simulink model "spmet_realtime"  (R2020a)
settings: Solver=FixedStepDiscrete  StartTime=0.0  StopTime=500  FixedStep=0.01  RelTol=1e-3  EnableMultiTasking=on
undefined symbols (not defined in the file or in its folder): Green, led0
libraries: simulink x1, embdlinuxlib x1
settings Model: Creator=Andreas  LastModifiedBy=Andreas
settings SolverCC: PositivePriorityOrder=on
settings OptimizationCC: EnhancedBackFolding=on  PassReuseOutputArgsAs=Individual arguments  ZeroExternalMemoryAtStartup=off  ZeroInternalMemoryAtStartup=off  MaxStackSize=64  OptimizeBlockOrder=speed  DifferentSizesBufferReuse=on  OptimizationCustomize=off  EfficientTunableParamExpr=on
settings DebuggingCC: ParameterTunabilityLossMsg=error  UnderSpecifiedDimensionMsg=warning
settings HardwareCC: ProdBitPerPointer=32  ProdBitPerSizeT=32  ProdBitPerPtrDiffT=32  ProdLargestAtomicInteger=Long  ProdLargestAtomicFloat=Double  ProdWordSize=32  ProdLongLongMode=on  ProdHWDeviceType=ARM Compatible->ARM Cortex
settings RTWCC: SystemTargetFile=ert.tlc  HardwareBoard=Raspberry Pi  TemplateMakefile=ert_default_tmf  GenerateReport=on  Toolchain=GNU GCC Raspberry Pi  BuildConfiguration=Faster Runs  IncludeHyperlinkInReport=on  LaunchReport=on  GenerateTraceInfo=on  GenerateTraceReport=on  GenerateTraceReportSl=on  GenerateTraceReportSf=on  GenerateTraceReportEml=on
settings CodeAppCC: ForceParamTrailComments=on  IgnoreCustomStorageClasses=off  OperatorAnnotations=on  SimulinkDataObjDesc=on  SFDataObjDesc=on  InsertBlockDesc=on
settings ERTTargetCC: SupportContinuousTime=on  SupportVariableSizeSignals=on

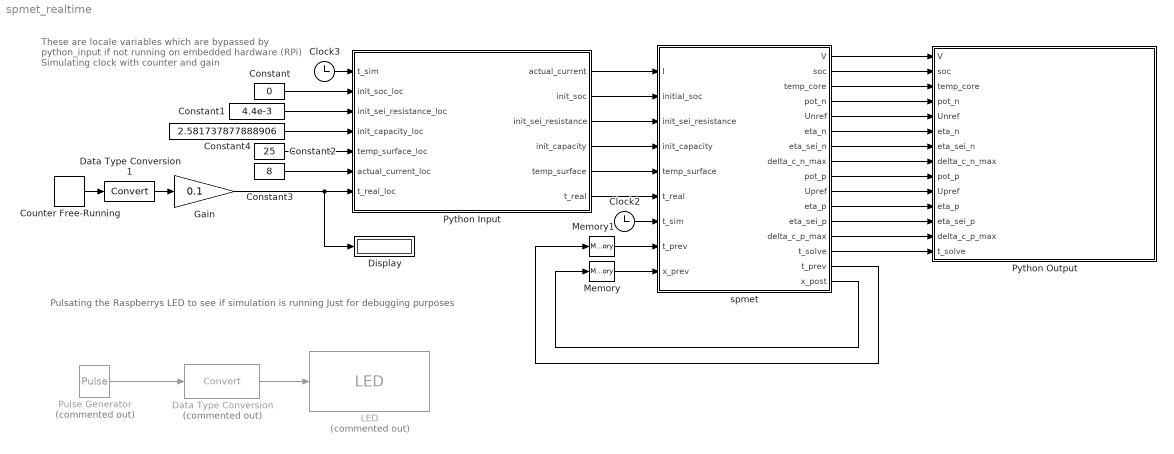
== system spmet_realtime ==
  note: Pulsating the Raspberrys LED to see if simulation is running
      | Just for debugging purposes
  note: These are locale variables
      | which are bypassed by
      | python_input if not running
      | on embedded hardware (RPi)
      |
      |
      |
      |
      |
      |
      |
      |
      | Simulating clock with counter and gain
  Clock2 : Clock
  Clock3 : Clock
  Constant : Constant  Value=0
  Constant1 : Constant  Value=4.4e-3
  Constant2 : Constant  Value=25
  Constant3 : Constant  Value=8
  Constant4 : Constant  Value=2.581737877888906
  Counter Free-Running : simulink/Sources/Counter Free-Running  NumBits=64  tsamp=-1
  Data Type Conversion : DataTypeConversion  Commented=on
  Data Type Conversion1 : DataTypeConversion
  Display : Display
  Gain : Gain  Gain=0.1
  LED : embdlinuxlib/LED  Commented=on  board=Pi 3 Model B+  led=led0 (Green)  blockPlatform=Raspberry Pi
      settings: SourceProductBaseCode=SC_BEAGLEBONE_BLUE,RASPPI
  Memory : Memory
  Memory1 : Memory
  Pulse Generator : DiscretePulseGenerator  Commented=on  PulseType=Time based  Period=4  PulseWidth=50
  Python Input : MATLAB Function  TreatAsAtomicUnit=on
  Python Output : MATLAB Function  TreatAsAtomicUnit=on
  spmet : MATLAB Function  TreatAsAtomicUnit=on
  wires:
  Data Type Conversion/1 -> LED/1
  Pulse Generator/1 -> Data Type Conversion/1
  Clock2/1 -> spmet/7(t_sim)
  Memory/1 -> spmet/9(x_prev)
  Memory1/1 -> spmet/8("t_prev ")
  Clock3/1 -> Python Input/1(t_sim)
  Python Input/2(init_soc) -> spmet/2(initial_soc)
  Python Input/1(actual_current) -> spmet/1(I)
  Constant/1 -> Python Input/2(init_soc_loc)
  Constant3/1 -> Python Input/6(actual_current_loc)
  Data Type Conversion1/1 -> Gain/1
  Counter Free-Running/1 -> Data Type Conversion1/1
  Gain/1 -> Display/1, Python Input/7(t_real_loc)
  spmet/16(x_post) -> Memory/1
  spmet/15(t_prev) -> Memory1/1
  Python Input/5(temp_surface) -> spmet/5(temp_surface)
  Python Input/6(t_real) -> spmet/6(t_real)
  Constant2/1 -> Python Input/5(temp_surface_loc)
  spmet/2(soc) -> Python Output/2(soc)
  spmet/3(temp_core) -> Python Output/3(temp_core)
  spmet/4(pot_n) -> Python Output/4(pot_n)
  spmet/5(Unref) -> Python Output/5(Unref)
  spmet/6(eta_n) -> Python Output/6(eta_n)
  spmet/7(eta_sei_n) -> Python Output/7(eta_sei_n)
  spmet/8(delta_c_n_max) -> Python Output/8(delta_c_n_max)
  spmet/9(pot_p) -> Python Output/9(pot_p)
  spmet/10(Upref) -> Python Output/10(Upref)
  spmet/11(eta_p) -> Python Output/11(eta_p)
  spmet/12(eta_sei_p) -> Python Output/12(eta_sei_p)
  spmet/13(delta_c_p_max) -> Python Output/13(delta_c_p_max)
  spmet/14(t_solve) -> Python Output/14(t_solve)
  spmet/1(V) -> Python Output/1(V)
  Python Input/4(init_capacity) -> spmet/4(init_capacity)
  Python Input/3(init_sei_resistance) -> spmet/3(init_sei_resistance)
  Constant1/1 -> Python Input/3(init_sei_resistance_loc)
  Constant4/1 -> Python Input/4(init_capacity_loc)

== matlab function spmet_realtime/Python Output ==
  data: V input; soc input; temp_core input; pot_n input; Unref input; eta_n input; eta_sei_n input; delta_c_n_max input; pot_p input; Upref input; eta_p input; eta_sei_p input; delta_c_p_max input; t_solve input
function python_output(V, soc, temp_core ,pot_n, Unref, eta_n, eta_sei_n, delta_c_n_max, pot_p, Upref, eta_p, eta_sei_p, delta_c_p_max, t_solve)
 
fprintf(1,"OUT_STRING: V=%f, soc=%f, temp_core=%f, pot_n=%f, Unref=%f, eta_n=%f, eta_sei_n=%f, delta_c_n_max=%f, pot_p=%f, Upref=%f, eta_p=%f, eta_sei_p=%f, delta_c_p_max=%f, t_solve=%f\n"...
            ,V,soc, temp_core, pot_n, Unref, eta_n, eta_sei_n, delta_c_n_max, pot_p, Upref, eta_p, eta_sei_p, delta_c_p_max, t_solve);

end

== matlab function spmet_realtime/Python Input ==
  data: actual_current output; init_soc output; init_sei_resistance output; init_capacity output; temp_surface output; t_sim input; t_real output; init_soc_loc input; init_sei_resistance_loc input; init_capacity_loc input; temp_surface_loc input; actual_current_loc input; t_real_loc input
function [actual_current, init_soc, init_sei_resistance, init_capacity, temp_surface, t_real]...
    =python_input(t_sim, init_soc_loc, init_sei_resistance_loc, init_capacity_loc, temp_surface_loc, actual_current_loc, t_real_loc)

if t_sim==0
    % at start of the Simulation
    
    fprintf(1,"init_soc\n");
    init_soc=0.0; %init
    init_soc=init_soc_loc; %setting to locale value
    coder.ceval('scanf','%lf',coder.ref(init_soc)); % read from stdin
    
    fprintf(1,"init_sei_resistance\n");
    init_sei_resistance=0.0; %init
    init_sei_resistance=init_sei_resistance_loc; %setting to locale value
    coder.ceval('scanf','%lf',coder.ref(init_sei_resistance)); % read from stdin
    
    fprintf(1,"init_capacity\n");
    init_capacity=0.0; %init
    init_capacity=init_capacity_loc; %setting to locale value
    coder.ceval('scanf','%lf',coder.ref(init_capacity)); % read from stdin

    
    % value is not used in first time step but the coder needs it defined
    actual_current=0;
    
else
    % during simulation
    fprintf(1,"actual_current\n");
    actual_current=0.0; %init
    actual_current=actual_current_loc; %setting to locale value
    coder.ceval('scanf','%lf',coder.ref(actual_current)); % read from stdin
    
    % value is not used in during simulation but the coder needs it defined
    init_soc=0;
    init_sei_resistance=0;
    init_capacity=0;

end

% needed in every time step

fprintf(1,"temp_surface\n");
temp_surface=0.0; %init
temp_surface=temp_surface_loc; %setting to locale value
coder.ceval('scanf','%lf',coder.ref(temp_surface)); % read from stdin

fprintf(1,"t_real\n");
t_real=0.0; %init
t_real=t_real_loc; %setting to locale value
coder.ceval('scanf','%lf',coder.ref(t_real)); % read from stdin
end

== matlab function spmet_realtime/spmet ==
  data: V output; soc output; temp_core output; pot_n output; Unref output; eta_n output; eta_sei_n output; delta_c_n_max output; pot_p output; Upref output; eta_p output; eta_sei_p output; delta_c_p_max output; t_solve output; I input; initial_soc input; init_sei_resistance input; init_capacity input; temp_surface input; t_real input; t_sim input; t_prev input; x_prev input; t_prev output; x_post output
function [V, soc, temp_core ,pot_n, Unref, eta_n, eta_sei_n, delta_c_n_max, pot_p, Upref, eta_p, eta_sei_p, delta_c_p_max, t_solve, t_prev, x_post]...
    = spmet(I, initial_soc, init_sei_resistance, init_capacity, temp_surface, t_real, t_sim, t_prev, x_prev)


%% Single Particle Model w/ Electrolyte & Temperature
% Published December 18, 2016 by Professor Scott Moura
% Adapted July 16, 2020 by Matthias Wanzel and Nikolaos Wassiliadis

% addpath(genpath(pwd));

%% Electrochemical model parameter
% Load US18650VTC5A NCA cell parameter
p = params_fn(init_capacity, init_sei_resistance);

%% Initial values for coder
% As the coder (for Simulink) needs to know the dimensions before
% assignment, the constant system matrices have to be defined here

p.ce.M1n = sparse(9,9);
p.ce.M2n = sparse(9,2);
p.ce.M3n = sparse(9,9);
p.ce.M4n = sparse(9,2);
p.ce.M5n = sparse(9,9);

p.ce.M1s = sparse(4,4);
p.ce.M2s = sparse(4,2);
p.ce.M3s = sparse(4,4);
p.ce.M4s = sparse(4,2);
p.ce.M1p = sparse(9,9);
p.ce.M2p = sparse(9,2);
p.ce.M3p = sparse(9,9);
p.ce.M4p = sparse(9,2);
p.ce.M5p = sparse(9,9);

p.ce.C = sparse(4,22);

% Calculate C-Rate
[cn_low,cp_low] = init_SOC(p,0);
[cn_high,cp_high] = init_SOC(p,100); 
Delta_cn = cn_high-cn_low;
Delta_cp = cp_low-cp_high;
qn = p.epsilon_s_n*p.Area*p.L_n*Delta_cn*p.Faraday/3600; 
qp = p.epsilon_s_p*p.Area*p.L_p*Delta_cp*p.Faraday/3600;
p.OneC = min(p.epsilon_s_n*p.L_n*Delta_cn*p.Area*p.Faraday/3600, p.epsilon_s_p*p.L_p*p.Area*Delta_cp*p.Faraday/3600);

%% Use one Input Value
% Live calculation based on Simulink input

if t_sim==0
    t_prev=t_real;
end

t_intermediate = (t_prev+t_real)/2;

t = [t_prev, t_intermediate, t_real];
I = I*ones(size(t));
T2 = temp_surface*ones(size(t));
t_prev = t_real;  

%% Input data structure with time, current and temperature
% Current | Positive <=> Charge | Negative <=> Discharge
data.time = t;          % [s]
data.cur = I;           % [A]
data.T2 = T2+273.15;    % [K]
NT = length(t);

%% Preallocation and initial conditions

% Finite difference for spherical particle
p.Nr = 20;
Nr = p.Nr;
p.delta_r_n = 1/p.Nr;
p.delta_r_p = 1/p.Nr;
r_vec = (0:p.delta_r_n:1)';
r_vecx = r_vec(2:end-1);

% Finite difference points along x-coordinate
p.Nxn = 10;
p.Nxs = 5;
p.Nxp = 10;
p.Nx = p.Nxn+p.Nxs+p.Nxp;
Nx = p.Nx - 3;
x_vec_spme = linspace(0,1,Nx+4);

p.delta_x_n = 1 / p.Nxn;
p.delta_x_s = 1 / p.Nxs;
p.delta_x_p = 1 / p.Nxp;

% Solid concentration
SOC_0 = initial_soc;
[csn0,csp0] = init_SOC(p,SOC_0);  
c_n0 = csn0 * ones(p.Nr-1,1);
c_p0 = csp0 * ones(p.Nr-1,1);

% Electrolyte concentration
ce0 = p.c_e*ones(Nx,1);

% Temperature
T10 = data.T2(1);

% SEI layer
delta_sei0 = 0;

%% Generate Constant System Matrices

% Electrolyte concentration matrices
[M1n,M2n,M3n,M4n,M5n, M1s,M2s,M3s,M4s, M1p,M2p,M3p,M4p,M5p, C_ce] = c_e_mats(p);

p.ce.M1n = M1n(1:9,1:9);
p.ce.M2n = M2n(1:9,1:2);
p.ce.M3n = M3n(1:9,1:9);
p.ce.M4n = M4n(1:9,1:2);
p.ce.M5n = M5n(1:9,1:9);

p.ce.M1s = M1s(1:4,1:4);
p.ce.M2s = M2s(1:4,1:2);
p.ce.M3s = M3s(1:4,1:4);
p.ce.M4s = M4s(1:4,1:2);

p.ce.M1p = M1p(1:9,1:9);
p.ce.M2p = M2p(1:9,1:2);
p.ce.M3p = M3p(1:9,1:9);
p.ce.M4p = M4p(1:9,1:2);
p.ce.M5p = M5p(1:9,1:9);

p.ce.C = C_ce(1:4,1:22);

% Differentiate between first (init) step and following simulation steps
if t_sim == 0
    %% Init when just startet (t=0)

    % Set old x vektor to the init x_0 vektor for the first simulation step
    x_post=[c_n0; c_p0; ce0; T10; delta_sei0];
    
    % Return output variables also at init (for simulink)
    V=0;
    pot_n=0;
    pot_p=0;
    soc=0;
    temp_core=0;
    Unref=0;
    eta_n=0;
    eta_sei_n=0;
    Upref=0;
    eta_p=0;
    eta_sei_p=0;
    delta_c_n_max=0;
    delta_c_p_max=0;
    t_solve=0;
else
    %% After initialization is done (t>0), simulate time step of SPMeT plant
    tic
    
    % calc x length = (particle count-surface)*2 + electrolyte + Temp + delta_sei)
    x_length=(p.Nr-1)*2+Nx+1+1;
    
    %using old x vektor as input for new simulation step
    x0 = x_prev;
    
    % Set Solver Parameters
    options = odeset('MaxStep',0.01);
    
    % Solver
    [t,x] = ode23(@(t,x) ode_spmet(t,x,data,p),t,x0,options);
    
    % extract only the lastest x-state (x has a time dimension of 3)
    x = x(NT,1:x_length);
    
    % Parse states   
    c_s_n = real(x(1:(p.Nr-1)));
    c_s_p = real(x(p.Nr : 2*(p.Nr-1)));
    c_e = real(x(2*p.Nr-1 : 2*p.Nr-1+p.Nx-4));
    T1 = real(x(end-1));
    delta_sei = real(x(end));
    
    x_post=x';

    %% Output Function for last t%%%
    V = 0.0;                % Voltage SPMeT
    V_spm = 0.0;            % Voltage without electrolyte
    SOC_n = 0.0;            % State of charge neg. electrode 
    SOC_p = 0.0;            % State of charge pos. electrode 
    c_ss_n = 0.0;           % Surface concentration neg. particle
    c_ss_p = 0.0;           % Surface concentration pos. particle
    c_e = zeros(p.Nx+1,1);  % Electrolyte concentrations
    eta_n = 0.0;            % Activation overpotential neg. electrode based on Butler–Volmer equation
    eta_p = 0.0;            % Activation overpotential pos. electrode based on Butler–Volmer equation
    Unref = 0.0;            % Equilibrium potential neg. electrode
    Upref = 0.0;            % Equilibrium potential pos. electrode
    V_ep = 0.0;             % Overpotential due to electrolyte polarization
    V_ec = 0.0;             % Overpotential due to electrolyte conductivity
    eta_sei_n = 0.0;        % Overpotential neg. electrode due to SEI resistance
    eta_sei_p = 0.0;        % Overpotential pos. electrode due to SEI resistance

    % Compute outputs 
    [~,V,V_spm,SOC_n,SOC_p,~,c_ss_p,c_e(:,1),eta_n,eta_p,Unref,Upref,V_ep,...
        V_ec, eta_sei_n, eta_sei_p, c_n, c_p] = ode_spmet(t(end),x_post,data,p);

    soc = soc_from_cell_state(p, SOC_p, SOC_n);
    pot_n=Unref + eta_n + eta_sei_n;
    pot_p=Upref+eta_p+eta_sei_p;
    temp_core=T1-273.15;
    
    % Calculation of max. diffusion gradient
    disp(c_p)
    delta_c_n_max=max(abs(gradient(c_n)))/(p.R_s_n*p.delta_r_n);
    disp(delta_c_n_max)
    
    delta_c_p_max=max(abs(gradient(c_p)))/(p.R_s_p*p.delta_r_p);
    disp(delta_c_p_max)
    

    % Output elapsed time
    t_solve = toc;
    disp('t_solve [ms]');
    disp(t_solve*1000);
end

end
